simulink model "bicycle"  (R2014b)
settings: Solver=ode45  StartTime=0.0  StopTime=200  RelTol=1e-3
values from neighbouring files (symbols this model uses):
  L = 2.5    [chassis_update.m]    (also in pure_pursuit_main.m = 10; pure_pursuit_main_dis.m = 10)
  velocity = 0.5    [pure_pursuit_main.m]    (also in pure_pursuit_main_dis.m)
settings Model: Creator=Bolin.zhao  LastModifiedBy=Administrator

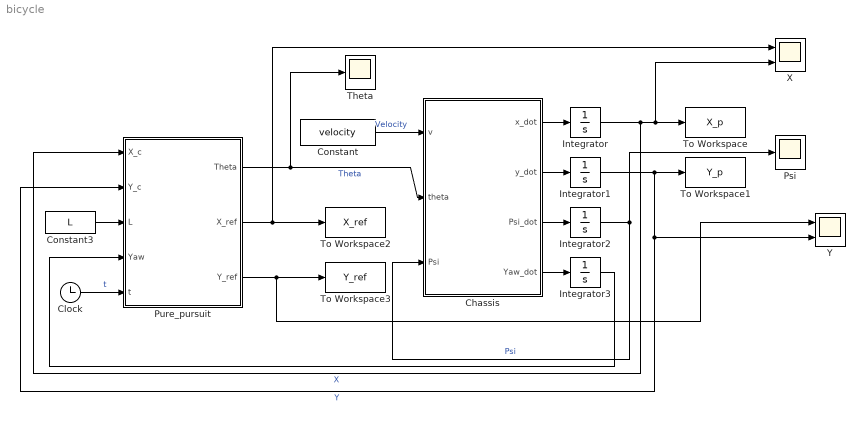
== system bicycle ==
  Chassis : MATLAB Function  TreatAsAtomicUnit=on
  Clock : Clock
  Constant : Constant  Value=velocity
  Constant3 : Constant  Value=L
  Integrator : Integrator  InitialCondition=3
  Integrator1 : Integrator
  Integrator2 : Integrator
  Integrator3 : Integrator
  Psi : Scope
      settings: SaveName=ScopeData2
  Pure_pursuit : MATLAB Function  TreatAsAtomicUnit=on
  Theta : Scope
      settings: SaveName=ScopeData3
  To Workspace : ToWorkspace  VariableName=X_p  SampleTime=-1
  To Workspace1 : ToWorkspace  VariableName=Y_p  SampleTime=-1
  To Workspace2 : ToWorkspace  VariableName=X_ref  SampleTime=-1
  To Workspace3 : ToWorkspace  VariableName=Y_ref  SampleTime=-1
  X : Scope  NumInputPorts=2
      settings: YMin=-5~-5  YMax=5~5
  Y : Scope  NumInputPorts=2
      settings: YMin=-5~-5  YMax=5~5
  wires:
  Constant/1 -> Chassis/1(v)  "Velocity"
  Chassis/1(x_dot) -> Integrator/1
  Chassis/2(y_dot) -> Integrator1/1
  Chassis/3(Psi_dot) -> Integrator2/1
  Integrator2/1 -> Chassis/3(Psi), Psi/1  "Psi"
  Integrator/1 -> Pure_pursuit/1(X_c), X/2, To Workspace/1  "X"
  Integrator1/1 -> Pure_pursuit/2(Y_c), Y/2, To Workspace1/1  "Y"
  Pure_pursuit/1(Theta) -> Chassis/2(theta), Theta/1  "Theta"
  Constant3/1 -> Pure_pursuit/3(L)
  Clock/1 -> Pure_pursuit/5(t)  "t"
  Pure_pursuit/2(X_ref) -> To Workspace2/1, X/1
  Pure_pursuit/3(Y_ref) -> To Workspace3/1, Y/1
  Chassis/4(Yaw_dot) -> Integrator3/1
  Integrator3/1 -> Pure_pursuit/4(Yaw)

== matlab function bicycle/Pure_pursuit ==
  data: X_c input; Theta output; Y_c input; L input; Yaw input; t input; X_ref output; Y_ref output
function [Theta, X_ref, Y_ref]   = Pure_pursuit( X_c, Y_c,L,  Yaw, t)
l =2.6; % wheelbase
%L = 1; % look ahead distance
X_ref = 20;%1*t;
Y_ref = 20;

P_e = sqrt((X_ref-X_c)^2 + (Y_ref - Y_c)^2);

p = polyfit([ X_c, X_ref], [Y_c, Y_ref],1);
if p(1) < 0 
     P_e = P_e*-1;% Turn right
end

Alfa = atan((Y_ref - Y_c)/(X_ref-X_c)) - Yaw;

%Theta = atan((2*l*P_e)/L^2);

Theta = atan((2*L*sin(Alfa))/l); %BJ GongYe Uni

if Theta > 1.5375 % constrain by the steering wheel
    Theta = 1.5375;
elseif Theta < -1.5375
   Theta = -1.5375;
end

return

== matlab function bicycle/Chassis ==
  data: v input; theta input; Psi input; x_dot output; y_dot output; Psi_dot output; Yaw_dot output
function [x_dot,y_dot, Psi_dot, Yaw_dot] = chassis_dynamics(v, theta, Psi)

l = 2.5;% wheelbase

x_dot = v*cos(Psi);
y_dot =v*sin(Psi);
Psi_dot = v*tan(theta)./l;
Yaw_dot = v/l*tan(Psi)

return
